simulink model "tutorial4"  (R2020a)
settings: Solver=FixedStepAuto  StartTime=0.0  StopTime=10.0  FixedStep=1e-3  RelTol=1e-3  EnableMultiTasking=on
libraries: dspstat3 x2
settings Model: ExtModeTrigDuration=5  Creator=qasim  LastModifiedBy=qasim
settings OptimizationCC: EnhancedBackFolding=on  PassReuseOutputArgsAs=Individual arguments  ZeroExternalMemoryAtStartup=off  ZeroInternalMemoryAtStartup=off  MaxStackSize=64  OptimizeBlockOrder=speed  DifferentSizesBufferReuse=on  OptimizationCustomize=off  EfficientTunableParamExpr=on
settings DebuggingCC: ParameterTunabilityLossMsg=error
settings HardwareCC: ProdBitPerPointer=32  ProdBitPerSizeT=32  ProdBitPerPtrDiffT=32  ProdLargestAtomicInteger=Long  ProdLargestAtomicFloat=Double  ProdWordSize=32  ProdHWDeviceType=ARM Compatible->ARM Cortex
settings SFSimCC: MATLABDynamicMemAlloc=off
settings RTWCC: SystemTargetFile=ert.tlc  HardwareBoard=NXP FRDM-K64F  TemplateMakefile=ert_default_tmf  Toolchain=GNU Tools for ARM Embedded Processors
settings CodeAppCC: ForceParamTrailComments=on  IgnoreCustomStorageClasses=off  OperatorAnnotations=on  SimulinkDataObjDesc=on  SFDataObjDesc=on  InsertBlockDesc=on

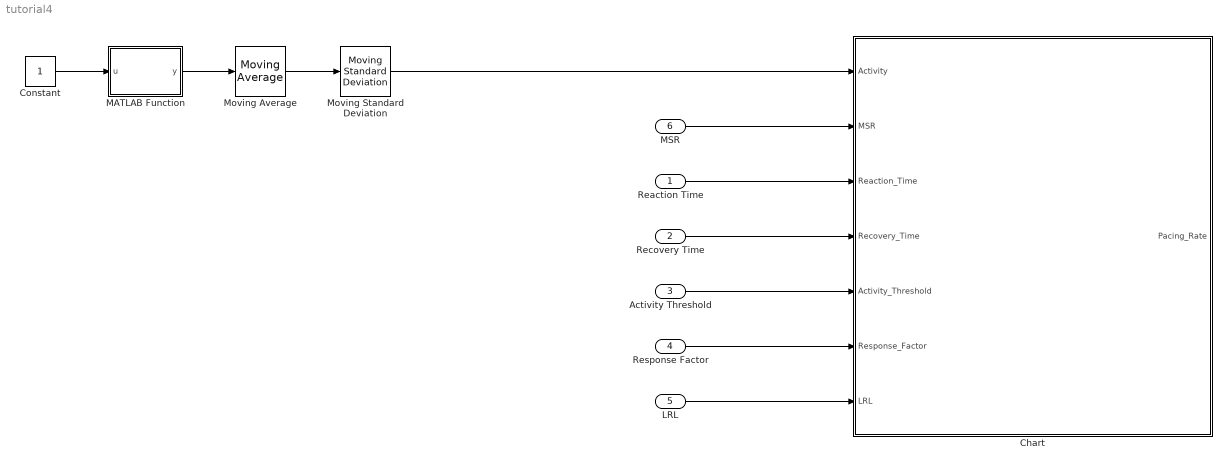
== system tutorial4 ==
  Reaction Time : Inport
  Recovery Time : Inport  Port=2
  Activity Threshold : Inport  Port=3
  Response Factor : Inport  Port=4
  LRL : Inport  Port=5
  MSR : Inport  Port=6
  Chart : Stateflow chart  TreatAsAtomicUnit=on
  Constant : Constant
  MATLAB Function : MATLAB Function  TreatAsAtomicUnit=on
  Moving Average : dspstat3/Moving Average  Method=Sliding window  ForgettingFactorPort=off  SpecifyWindowLength=on  WindowLength=10  ForgettingFactor=0.9  SimulateUsing=Code generation
  Moving Standard Deviation : dspstat3/Moving Standard Deviation  Method=Sliding window  ForgettingFactorPort=off  SpecifyWindowLength=on  WindowLength=10  ForgettingFactor=0.9  SimulateUsing=Code generation
      settings: SourceProductBaseCode=DS
  wires:
  Constant/1 -> MATLAB Function/1(u)
  MATLAB Function/1(y) -> Moving Average/1
  Moving Average/1 -> Moving Standard Deviation/1
  Moving Standard Deviation/1 -> Chart/1(Activity)
  Recovery Time/1 -> Chart/4(Recovery_Time)
  Reaction Time/1 -> Chart/3(Reaction_Time)
  Activity Threshold/1 -> Chart/5(Activity_Threshold)
  Response Factor/1 -> Chart/6(Response_Factor)
  LRL/1 -> Chart/7(LRL)
  MSR/1 -> Chart/2(MSR)

== matlab function tutorial4/MATLAB Function ==
  data: u input; y output
function y = fcn(u)

y = sqrt(u(1)^2+u(2)^2+u(3)^2);

== stateflow chart tutorial4/Chart ==
  state Start
    entry:
    Pacing_Rate = LRL;
    Time = 0;
  state Increase_Rate
    entry:
    Time = 0;
    target =(((MSR-LRL)/16)*Response_Factor*Activity)+LRL;
    step_up = (target-LRL)/Reaction_Time;
    during:
    Pacing_Rate = Pacing_Rate + step_up;
    Time = Time + 1/1000;
    exit:
    Time = 0;
  state Decrease_Rate
    entry:
    Time = 0;
    target =(((MSR-LRL)/16)*Response_Factor*Activity)+LRL;
    step_down = (target-LRL)/Recovery_Time;
    during:
    Pacing_Rate = Pacing_Rate-step_down;
    Time = Time + 1;
    exit:
    Time = 0;
  state Rate_above_LRL
    entry:
    Pacing_Rate = MSR;
  state Rate_below_LRL
    entry:
    Pacing_Rate = LRL;
  (default) -> Start
  Start -> Increase_Rate [order 1] : [Activity <= Activity_Threshold]
  Start -> Decrease_Rate [order 2] : [Activity > Activity_Threshold]
  Decrease_Rate -> Decrease_Rate [order 1] : [Time > Recovery_Time]{Time = 0}
  Increase_Rate -> Increase_Rate [order 1] : [Time > Reaction_Time]{Time = 0}
  Increase_Rate -> Decrease_Rate [order 2] : [Activity > Activity_Threshold]
  Decrease_Rate -> Increase_Rate [order 3] : [Activity <= Activity_Threshold]
  Decrease_Rate -> Rate_above_LRL [order 2] : [Pacing_Rate >= MSR]
  Rate_above_LRL -> Decrease_Rate
  Increase_Rate -> Rate_below_LRL [order 3] : [Pacing_Rate < LRL]
  Rate_below_LRL -> Increase_Rate
  data: Activity input; MSR input; Reaction_Time input; Recovery_Time input; Activity_Threshold input; Response_Factor input; LRL input; Pacing_Rate output; Time local; step_down local; step_up local; target local
